simulink library "StateMachine"  (R2025a)
settings: Solver=VariableStepAuto  StartTime=0.0  StopTime=10.0  RelTol=1e-3
values from neighbouring files (symbols this model uses):
  VehicleState : value not decoded    [StateMachine.sldd]
undefined symbols (not defined in the file or in its folder): dt
libraries: simulink x2, Utilities x1
settings Model: RaptorUIDSize=4  Creator=serga  LastModifiedBy=hyuga

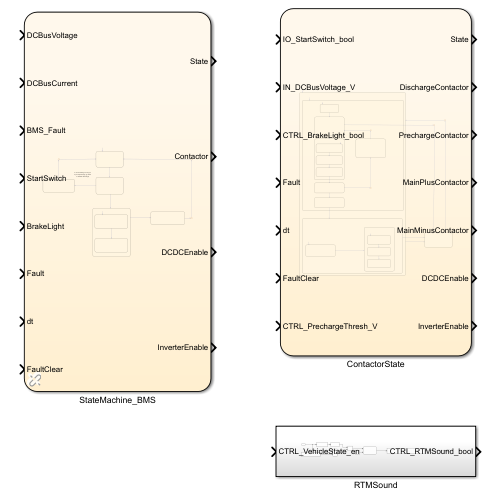
[thumbnail: Simulink's stored preview of the top-level diagram]
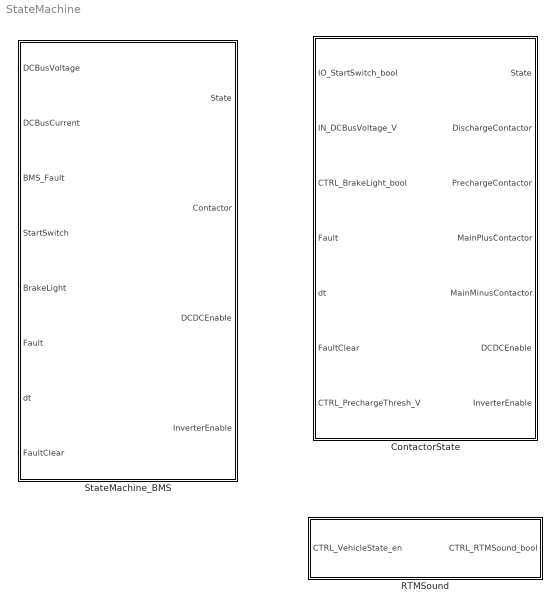
== system StateMachine ==
  ContactorState : Stateflow chart  TreatAsAtomicUnit=on
  RTMSound : Subsystem
  StateMachine_BMS : Stateflow chart  AncestorBlock=StateMachine/StateMachine_BMS  TreatAsAtomicUnit=on

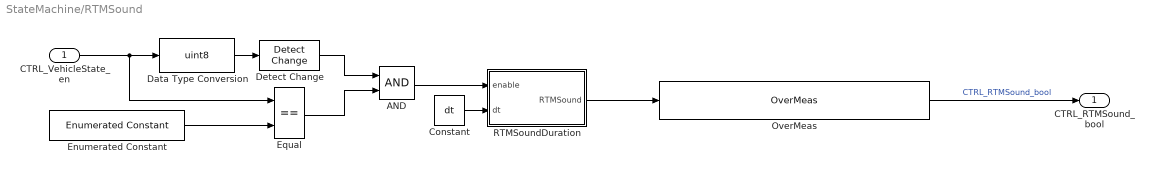
== system StateMachine/RTMSound ==
  CTRL_VehicleState_en : Inport
  AND : Logic  AllPortsSameDT=off  OutDataTypeStr=boolean
  Constant : Constant  Value=dt
  Data Type Conversion : DataTypeConversion  OutDataTypeStr=uint8  SaturateOnIntegerOverflow=off  RndMeth=Floor
  Detect Change : simulink/Logic and Bit Operations/Detect Change  vinit=0  OutDataTypeStr=boolean
  Enumerated Constant : simulink/Sources/Enumerated Constant  OutDataTypeStr=Enum: VehicleState  Value=VehicleState.ReadyToMove  SampleTime=inf
  Equal : RelationalOperator  Operator===  OutDataTypeStr=boolean  RndMeth=Simplest  InputSameDT=off
  OverMeas : Utilities/OverMeas  sigName='CTRL_RTMSound_bool'  minimum=0  maximum=1
  RTMSoundDuration : Stateflow chart  TreatAsAtomicUnit=on
  CTRL_RTMSound_bool : Outport
  wires:
  OverMeas/1 -> CTRL_RTMSound_bool/1  "CTRL_RTMSound_bool"
  Detect Change/1 -> AND/1
  Enumerated Constant/1 -> Equal/2
  CTRL_VehicleState_en/1 -> Data Type Conversion/1, Equal/1
  Data Type Conversion/1 -> Detect Change/1
  Equal/1 -> AND/2
  AND/1 -> RTMSoundDuration/1(enable)
  Constant/1 -> RTMSoundDuration/2(dt)
  RTMSoundDuration/1(RTMSound) -> OverMeas/1

== stateflow chart StateMachine/StateMachine_BMS ==
  state Default_Discharge
    entry:
    timer = 0;
    State = VehicleState.Default;
    Contactor = ContactorFault.NoFault;
    DCDCEnable = DCDCStatus.Off;
    InverterEnable = InverterStatus.Off;
    during:
    timer = timer + dt;
  note: if we are taking too long to try and precharge, go back to default/ discharge
  state Precharge
    entry:
    timer = 0;
    State = VehicleState.Precharge;
    Contactor = ContactorFault.NoFault;
    DCDCEnable = DCDCStatus.Off;
    InverterEnable = InverterStatus.Off;
    during:
    timer = timer + dt
  state PrechargeFault
    entry:
    State = VehicleState.PrechargeFault;
    Contactor = ContactorFault.PrechargeFault;
    DCDCEnable = DCDCStatus.Off;
    InverterEnable = InverterStatus.Off;
  state ReadyToMove
    state Standby
      entry:
      State = VehicleState.PrechargeComplete;
      Contactor = ContactorFault.NoFault;
      DCDCEnable = DCDCStatus.Off;
      InverterEnable = InverterStatus.Off;
    state RTM
      entry:
      State = VehicleState.ReadyToMove;
      Contactor = ContactorFault.NoFault;
      DCDCEnable = DCDCStatus.On;
      InverterEnable = InverterStatus.On;
    (default) -> Standby
    Standby -> RTM : [Fault == 0 ...
        | && BMS_Fault == 0 ...
        | && BrakeLight == 1 ...
        | && StartSwitch == 1]
  state ReadyToMoveFault
    entry:
    State = VehicleState.ReadyToMoveFault;
    Contactor = ContactorFault.ReadyToMoveFault;
    DCDCEnable = DCDCStatus.Off;
    InverterEnable = InverterStatus.Off;
  (default) -> Default_Discharge
  (junction 38) -> Default_Discharge
  (junction 47) -> Default_Discharge
  PrechargeFault -> (junction 38)
  (junction 45) -> (junction 47)
  Default_Discharge -> Precharge : [timer > 500 ...
      | && Fault == 0 ...
      | && BMS_Fault == 0]
  Precharge -> PrechargeFault [order 1] : [Fault == 1 ...
      | && timer > 500]
  Precharge -> ReadyToMove [order 2] : [Fault == 0 ...
      | && BMS_Fault == 0 ...
      | && DCBusCurrent <= 5 ...
      | && DCBusCurrent >= 0 ...
      | && DCBusVoltage >= 270]
  ReadyToMove -> ReadyToMoveFault : [Fault == 1 ...
      | && BMS_Fault == 1]
  ReadyToMoveFault -> (junction 45)
  data: State output; Contactor output; DCBusVoltage input; DCBusCurrent input; BMS_Fault input; StartSwitch input; BrakeLight input; Fault input; dt input; FaultClear input; DCDCEnable output; timer local uint32; InverterEnable output

== stateflow chart StateMachine/RTMSound/RTMSoundDuration ==
  state RTMSoundStop
    en:
    RTMSound = false;
    timer = 0;
  state RTMSoundStart
    en:
    RTMSound = true;
    du:
    timer = timer + dt;
  (default) -> RTMSoundStop
  RTMSoundStop -> RTMSoundStart : [enable == true]
  RTMSoundStart -> RTMSoundStop : [timer > 200]
  data: RTMSound output =false; enable input; timer local single; dt input

== stateflow chart StateMachine/ContactorState ==
  state Normal
    state Precharge
      state StartDelay
        en:
        timer = 0;
        State = VehicleState.StartDelay;
        du:
        timer = timer + dt;
      note: if there is already accumulator voltage present before even actuating the contactors, then a contactor has been welded
      state PrechargeReady
        % waiting for tractive system switch signal
        en:
        State = VehicleState.PrechargeReady;
        MainPlusContactor = ContactorState.Open;
        MainMinusContactor = ContactorState.Open;
        PrechargeContactor = ContactorState.Open;
        DischargeContactor = ContactorState.Close;
        DCDCEnable = DCDCStatus.Off;
        InverterEnable = InverterStatus.Off;
        timer = 0;
        du:
        timer = timer + dt;
      note: about 1 sec to discharge to 60V
      state PrechargeBegin
        en:
        State = VehicleState.Precharge;
        state DischargeDisable
          en:
          DischargeContactor = ContactorState.Open;
          timer = 0;
          du:
          timer = timer + dt;
        state PrechargeEnable
          en:
          PrechargeContactor = ContactorState.Close;
          timer = 0;
          du:
          timer = timer + dt;
        state MainMinusEnable
          en:
          MainMinusContactor = ContactorState.Close;
          timer = 0;
          du:
          timer = timer + dt;
        (default) -> DischargeDisable
        DischargeDisable -> PrechargeEnable : [timer >  50]
        PrechargeEnable -> MainMinusEnable : [timer >  50]
      state PrechargeTimeout
        % timed out, retry
        en:
        State = VehicleState.PrechargeTimeout
        MainPlusContactor = ContactorState.Open;
        MainMinusContactor = ContactorState.Open;
        PrechargeContactor = ContactorState.Open;
        DischargeContactor = ContactorState.Close;
        DCDCEnable = DCDCStatus.Off;
        InverterEnable = InverterStatus.Off;
        timer = 0;
        du:
        timer = timer + dt;
      note: change to something else -- this is just for testing
      state PrechargeWait
        % after closing the contactor, start the precharge timer
        du:
        timer = timer + dt;
      state PrechargeComplete
        en:
        State = VehicleState.PrechargeComplete;
        timer = 0;
      (default) -> StartDelay
      StartDelay -> PrechargeReady : [timer >  500 ...
          | && Fault == false]
      (junction 38) -> PrechargeReady
      PrechargeTimeout -> (junction 38) : [timer >  500]
      PrechargeReady -> PrechargeBegin [order 2] : [timer > 50]
      (junction 27) -> PrechargeTimeout
      MainMinusEnable -> PrechargeWait : [timer >  50]
      PrechargeWait -> (junction 27) [order 2] : [timer >  15000]
      PrechargeWait -> PrechargeComplete [order 1] : [IN_DCBusVoltage_V > CTRL_PrechargeThresh_V]
    state ReadyToMove
      state RTM
        en:
        State = VehicleState.ReadyToMove;
        state PrechargeDisable
          en:
          PrechargeContactor = ContactorState.Open;
          timer = 0;
          du:
          timer = timer + dt;
        state MainPlusEnable
          en:
          MainPlusContactor = ContactorState.Close;
          timer = 0;
          du:
          timer = timer + dt;
        state SpinUp
          en:
          InverterEnable = InverterStatus.On;
          DCDCEnable = DCDCStatus.On;
          timer = 0;
        (default) -> PrechargeDisable
        PrechargeDisable -> MainPlusEnable : [timer > 50]
        MainPlusEnable -> SpinUp : [timer > 50]
      state Standby
        % wait for all conditions to be satisfied
        en:
        State = VehicleState.Standby;
        du:
        timer = timer + dt;
      (default) -> Standby
      Standby -> RTM : [DischargeContactor == ContactorState.Open ...
          | && PrechargeContactor == ContactorState.Close ...
          | && MainMinusContactor == ContactorState.Close ...
          | && CTRL_BrakeLight_bool == true ...
          | && IO_StartSwitch_bool == true]
    (default) -> Precharge
    PrechargeComplete -> ReadyToMove : [DischargeContactor == ContactorState.Open ...
        | && MainMinusContactor == ContactorState.Close]
  note: watch for voltage sag
  state Faulted
    en:
    State = VehicleState.Faulted;
    MainPlusContactor = ContactorState.Open;
    MainMinusContactor = ContactorState.Open;
    PrechargeContactor = ContactorState.Open;
    DischargeContactor = ContactorState.Close;
    DCDCEnable = DCDCStatus.Off;
    InverterEnable = InverterStatus.Off;
    timer = 0;
  (default) -> Normal
  (junction 119) -> Normal
  Faulted -> (junction 119)
  PrechargeReady -> (junction 104) [order 1] : [duration(IN_DCBusVoltage_V > 60) > 2]
  (junction 104) -> Faulted
  ReadyToMove -> Faulted : [IN_DCBusVoltage_V < 210 ...
      | || IN_DCBusVoltage_V > 405]
  Normal -> Faulted : [Fault == true]
  data: State output; IO_StartSwitch_bool input; DischargeContactor output; PrechargeContactor output; MainPlusContactor output; MainMinusContactor output; timer local single; IN_DCBusVoltage_V input; CTRL_BrakeLight_bool input; Fault input; dt input; DCDCEnable output; InverterEnable output; FaultClear input; CTRL_PrechargeThresh_V input
